simulink model "problem17"  (R2021a)
settings: Solver=VariableStepAuto  StartTime=0.0  StopTime=8  RelTol=1e-3
undefined symbols (not defined in the file): a4, B, d1, J1, J2, J3, J4, Kd_1, Kd_2, Kd_3, Kd_4, Ki_1, Ki_2, Ki_3, Ki_4, Kp_1, Kp_2, Kp_3, Kp_4, n, T1, T2, T3, T4
settings Model: Creator=kays_  LastModifiedBy=Luky

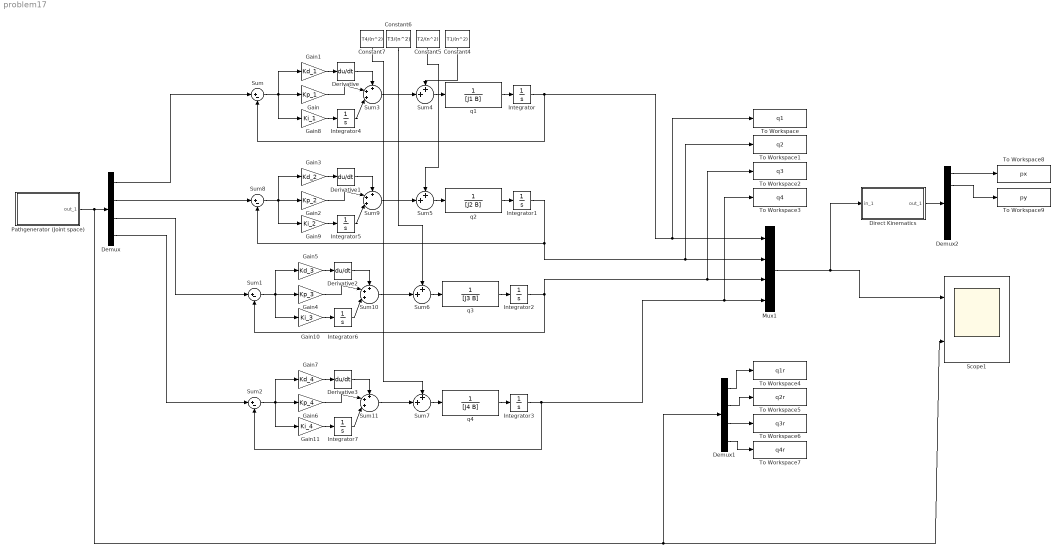
== system problem17 ==
  Constant4 : Constant  Value=T1/(n^2)
  Constant5 : Constant  Value=T2/(n^2)
  Constant6 : Constant  Value=T3/(n^2)
  Constant7 : Constant  Value=T4/(n^2)
  Demux : Demux
  Demux1 : Demux
  Demux2 : Demux  Outputs=6
  Derivative{,1..3} (4 alike) : Derivative
  Direct Kinematics : Subsystem
      mask Display: disp('Alto-Robot')
  Gain : Gain  Gain=Kp_1
  Gain1 : Gain  Gain=Kd_1
  Gain10 : Gain  Gain=Ki_3
  Gain11 : Gain  Gain=Ki_4
  Gain2 : Gain  Gain=Kp_2
  Gain3 : Gain  Gain=Kd_2
  Gain4 : Gain  Gain=Kp_3
  Gain5 : Gain  Gain=Kd_3
  Gain6 : Gain  Gain=Kp_4
  Gain7 : Gain  Gain=Kd_4
  Gain8 : Gain  Gain=Ki_1
  Gain9 : Gain  Gain=Ki_2
  Integrator{,1..7} (8 alike) : Integrator
  Mux1 : Mux
  Pathgenerator (Joint space) : Subsystem
      mask Display: disp('Alto-Robot\n path -> q')
  Scope1 : Scope  NumInputPorts=2
  Sum{,1..2,8} (4 alike) : Sum  Inputs=|+-
  Sum{3,9..11} (4 alike) : Sum  Inputs=+++|
  Sum{4..7} (4 alike) : Sum  Inputs=++|
  To Workspace : ToWorkspace  VariableName=q1  SaveFormat=Timeseries  SampleTime=-1
  To Workspace1 : ToWorkspace  VariableName=q2  SaveFormat=Timeseries  SampleTime=-1
  To Workspace2 : ToWorkspace  VariableName=q3  SaveFormat=Timeseries  SampleTime=-1
  To Workspace3 : ToWorkspace  VariableName=q4  SaveFormat=Timeseries  SampleTime=-1
  To Workspace4 : ToWorkspace  VariableName=q1r  SaveFormat=Timeseries  SampleTime=-1
  To Workspace5 : ToWorkspace  VariableName=q2r  SaveFormat=Timeseries  SampleTime=-1
  To Workspace6 : ToWorkspace  VariableName=q3r  SaveFormat=Timeseries  SampleTime=-1
  To Workspace7 : ToWorkspace  VariableName=q4r  SaveFormat=Timeseries  SampleTime=-1
  To Workspace8 : ToWorkspace  VariableName=px  SaveFormat=Timeseries  SampleTime=-1
  To Workspace9 : ToWorkspace  VariableName=py  SaveFormat=Timeseries  SampleTime=-1
  q1 : TransferFcn  Denominator=[J1 B]
  q2 : TransferFcn  Denominator=[J2 B]
  q3 : TransferFcn  Denominator=[J3 B]
  q4 : TransferFcn  Denominator=[J4 B]
  wires:
  Sum7/1 -> q4/1
  Sum/1 -> Gain8/1, Gain1/1, Gain/1
  Gain/1 -> Sum3/2
  Gain3/1 -> Derivative1/1
  Demux/2 -> Sum8/1
  q4/1 -> Integrator3/1
  Demux/1 -> Sum/1
  Sum5/1 -> q2/1
  Integrator4/1 -> Sum3/3
  Sum9/1 -> Sum5/2
  Gain10/1 -> Integrator6/1
  Gain11/1 -> Integrator7/1
  Integrator/1 -> To Workspace/1, Mux1/1, Sum/2
  Sum11/1 -> Sum7/2
  Integrator7/1 -> Sum11/3
  Sum4/1 -> q1/1
  Gain5/1 -> Derivative2/1
  Gain2/1 -> Sum9/2
  Integrator5/1 -> Sum9/3
  Gain8/1 -> Integrator4/1
  Gain7/1 -> Derivative3/1
  q3/1 -> Integrator2/1
  Sum3/1 -> Sum4/2
  Derivative3/1 -> Sum11/1
  Gain1/1 -> Derivative/1
  q1/1 -> Integrator/1
  Derivative1/1 -> Sum9/1
  Gain9/1 -> Integrator5/1
  q2/1 -> Integrator1/1
  Gain6/1 -> Sum11/2
  Integrator1/1 -> To Workspace1/1, Mux1/2, Sum8/2
  Derivative2/1 -> Sum10/1
  Sum2/1 -> Gain11/1, Gain7/1, Gain6/1
  Integrator6/1 -> Sum10/3
  Integrator2/1 -> Sum1/2, To Workspace2/1, Mux1/3
  Sum1/1 -> Gain10/1, Gain5/1, Gain4/1
  Integrator3/1 -> To Workspace3/1, Mux1/4, Sum2/2
  Gain4/1 -> Sum10/2
  Sum6/1 -> q3/1
  Derivative/1 -> Sum3/1
  Sum10/1 -> Sum6/2
  Sum8/1 -> Gain9/1, Gain3/1, Gain2/1
  Demux/3 -> Sum1/1
  Demux/4 -> Sum2/1
  Mux1/1 -> Direct Kinematics/1(in_1), Scope1/1
  Pathgenerator (Joint space)/1(out_1) -> Demux1/1, Scope1/2, Demux/1
  Demux1/1 -> To Workspace4/1
  Demux1/2 -> To Workspace5/1
  Demux1/3 -> To Workspace6/1
  Demux1/4 -> To Workspace7/1
  Direct Kinematics/1(out_1) -> Demux2/1
  Demux2/1 -> To Workspace8/1
  Demux2/2 -> To Workspace9/1
  Constant6/1 -> Sum6/1
  Constant7/1 -> Sum7/1
  Constant5/1 -> Sum5/1
  Constant4/1 -> Sum4/1

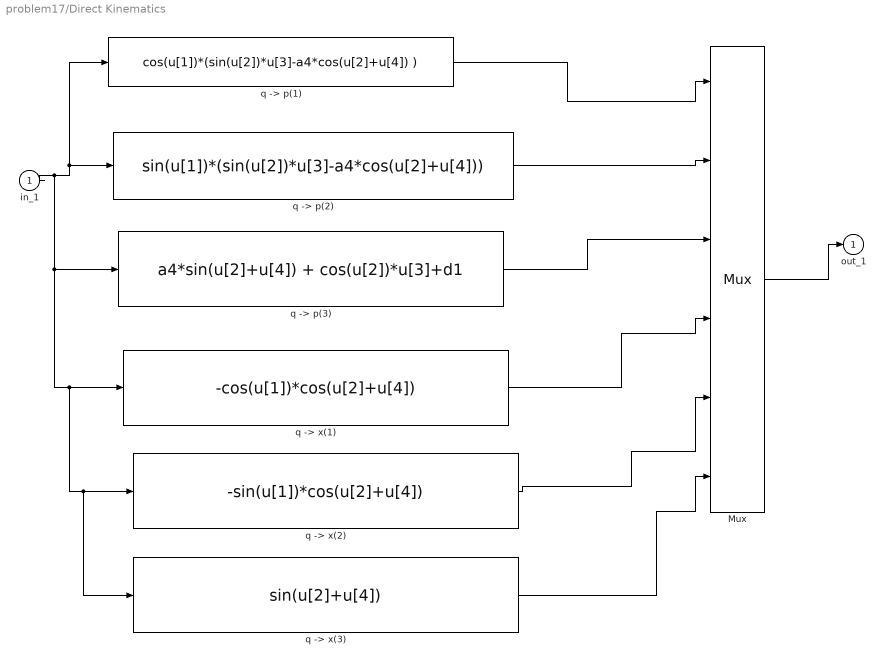
== system problem17/Direct Kinematics ==
  in_1 : Inport
  Mux : Mux  Inputs=6
  "q -> p(1)" : Fcn  Expr=cos(u[1])*(sin(u[2])*u[3]-a4*cos(u[2]+u[4]) )
  "q -> p(2)" : Fcn  Expr=sin(u[1])*(sin(u[2])*u[3]-a4*cos(u[2]+u[4]))
  "q -> p(3)" : Fcn  Expr=a4*sin(u[2]+u[4]) + cos(u[2])*u[3]+d1
  "q -> x(1)" : Fcn  Expr=-cos(u[1])*cos(u[2]+u[4])
  "q -> x(2)" : Fcn  Expr=-sin(u[1])*cos(u[2]+u[4])
  "q -> x(3)" : Fcn  Expr=sin(u[2]+u[4])
  out_1 : Outport  InitialOutput=0  VectorParamsAs1DForOutWhenUnconnected=off
  wires:
  Mux/1 -> out_1/1
  in_1/1 -> "q -> x(3)"/1, "q -> x(2)"/1, "q -> x(1)"/1, "q -> p(3)"/1, "q -> p(2)"/1, "q -> p(1)"/1
  "q -> x(3)"/1 -> Mux/6
  "q -> x(2)"/1 -> Mux/5
  "q -> x(1)"/1 -> Mux/4
  "q -> p(1)"/1 -> Mux/1
  "q -> p(2)"/1 -> Mux/2
  "q -> p(3)"/1 -> Mux/3

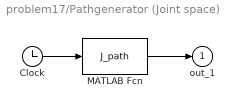
== system problem17/Pathgenerator (Joint space) ==
  Clock : Clock
  MATLAB Fcn : MATLABFcn  MATLABFcn=J_path  OutputDimensions=4
  out_1 : Outport  VectorParamsAs1DForOutWhenUnconnected=off
  wires:
  MATLAB Fcn/1 -> out_1/1
  Clock/1 -> MATLAB Fcn/1
